simulink model "compute_control"  (R2020a)
settings: Solver=VariableStepAuto  StartTime=0.0  StopTime=0.7  RelTol=1e-3
values from neighbouring files (symbols this model uses):
  A = [-b_cv/Je, 0, -k/Je;     -b_cv/Je+b_ck/Jeq, -b_ck/Jeq, -(k/Je+k/Jeq);     0 0 0]    [Parameters.m]
  B = [0;0;1]    [Parameters.m]
  Gamma = Bd*d    [Parameters.m]
  Q = [0, 0,    0;     0,  50000, 0;     0,  0,    0]    [Parameters.m]
  R = 1    [Parameters.m]
settings Model: Creator=andre  LastModifiedBy=andre

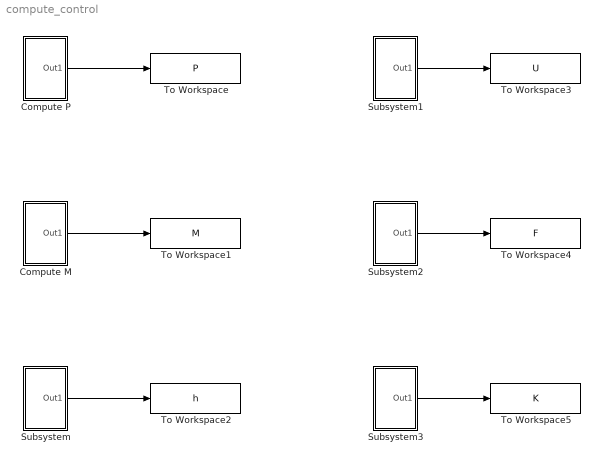
== system compute_control ==
  Compute M : Subsystem
  Compute P : Subsystem
  Subsystem : Subsystem
  Subsystem1 : Subsystem
  Subsystem2 : Subsystem
  Subsystem3 : Subsystem
  To Workspace : ToWorkspace  VariableName=P  SampleTime=-1
  To Workspace1 : ToWorkspace  VariableName=M  SampleTime=-1
  To Workspace2 : ToWorkspace  VariableName=h  SampleTime=-1
  To Workspace3 : ToWorkspace  VariableName=U  SampleTime=-1
  To Workspace4 : ToWorkspace  VariableName=F  SampleTime=-1
  To Workspace5 : ToWorkspace  VariableName=K  SampleTime=-1
  wires:
  Compute P/1(Out1) -> To Workspace/1
  Compute M/1(Out1) -> To Workspace1/1
  Subsystem/1(Out1) -> To Workspace2/1
  Subsystem1/1(Out1) -> To Workspace3/1
  Subsystem2/1(Out1) -> To Workspace4/1
  Subsystem3/1(Out1) -> To Workspace5/1

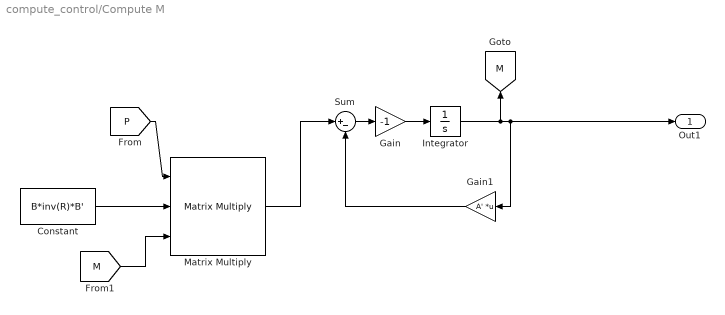
== system compute_control/Compute M ==
  Constant : Constant  Value=B*inv(R)*B'
  Gain : Gain  Gain=-1
  Gain1 : Gain  Gain=A'  Multiplication=Matrix(K*u)
  Integrator : Integrator  InitialCondition=[0;1;0]
  Matrix Multiply : Product  Inputs=3  Multiplication=Matrix(*)
  Sum : Sum  Inputs=|+-
  Out1 : Outport
  tag scope: M=global
  wires:
  [P] -> Matrix Multiply/1
  Gain1/1 -> Sum/2
  Sum/1 -> Gain/1
  Gain/1 -> Integrator/1
  Matrix Multiply/1 -> Sum/1
  Constant/1 -> Matrix Multiply/2
  Integrator/1 -> [M], Out1/1, Gain1/1
  [M] -> Matrix Multiply/3

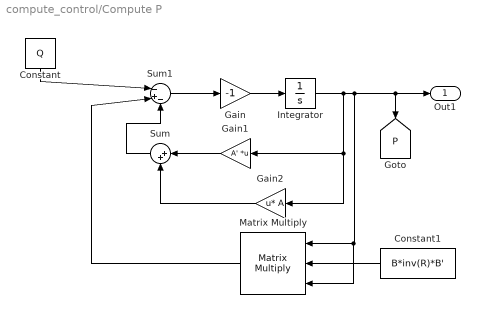
== system compute_control/Compute P ==
  Constant : Constant  Value=Q
  Constant1 : Constant  Value=B*inv(R)*B'
  Gain : Gain  Gain=-1
  Gain1 : Gain  Gain=A'  Multiplication=Matrix(K*u)
  Gain2 : Gain  Gain=A  Multiplication=Matrix(u*K)
  Integrator : Integrator  InitialCondition=zeros(3,3)
  Matrix Multiply : Product  Inputs=3  Multiplication=Matrix(*)
  Sum : Sum  Inputs=|++
  Sum1 : Sum  Inputs=|-+-
  Out1 : Outport
  tag scope: P=global
  wires:
  Sum/1 -> Sum1/3
  Integrator/1 -> Gain1/1, Gain2/1, [P], Out1/1, Matrix Multiply/3, Matrix Multiply/1
  Sum1/1 -> Gain/1
  Constant/1 -> Sum1/1
  Gain/1 -> Integrator/1
  Gain2/1 -> Sum/2
  Gain1/1 -> Sum/1
  Matrix Multiply/1 -> Sum1/2
  Constant1/1 -> Matrix Multiply/2

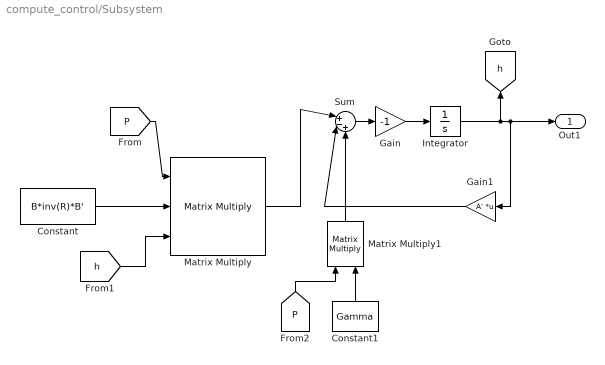
== system compute_control/Subsystem ==
  Constant : Constant  Value=B*inv(R)*B'
  Constant1 : Constant  Value=Gamma
  Gain : Gain  Gain=-1
  Gain1 : Gain  Gain=A'  Multiplication=Matrix(K*u)
  Integrator : Integrator  InitialCondition=[0;0;0]
  Matrix Multiply : Product  Inputs=3  Multiplication=Matrix(*)
  Matrix Multiply1 : Product  Multiplication=Matrix(*)
  Sum : Sum  Inputs=|+-+
  Out1 : Outport
  tag scope: h=global
  wires:
  [h] -> Matrix Multiply/3
  Constant/1 -> Matrix Multiply/2
  Integrator/1 -> [h], Out1/1, Gain1/1
  Gain/1 -> Integrator/1
  Sum/1 -> Gain/1
  Gain1/1 -> Sum/2
  [P] -> Matrix Multiply1/1
  Matrix Multiply/1 -> Sum/1
  [P] -> Matrix Multiply/1
  Matrix Multiply1/1 -> Sum/3
  Constant1/1 -> Matrix Multiply1/2

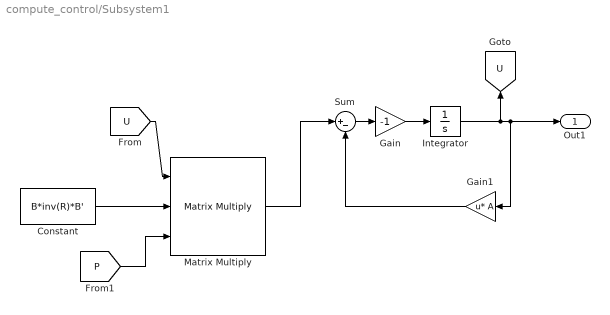
== system compute_control/Subsystem1 ==
  Constant : Constant  Value=B*inv(R)*B'
  Gain : Gain  Gain=-1
  Gain1 : Gain  Gain=A  Multiplication=Matrix(u*K)
  Integrator : Integrator  InitialCondition=[0 1 0]
  Matrix Multiply : Product  Inputs=3  Multiplication=Matrix(*)
  Sum : Sum  Inputs=|+-
  Out1 : Outport
  tag scope: U=global
  wires:
  Gain/1 -> Integrator/1
  Gain1/1 -> Sum/2
  Matrix Multiply/1 -> Sum/1
  Constant/1 -> Matrix Multiply/2
  [P] -> Matrix Multiply/3
  Sum/1 -> Gain/1
  Integrator/1 -> [U], Out1/1, Gain1/1
  [U] -> Matrix Multiply/1

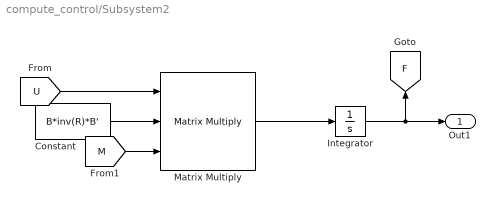
== system compute_control/Subsystem2 ==
  Constant : Constant  Value=B*inv(R)*B'
  Integrator : Integrator
  Matrix Multiply : Product  Inputs=3  Multiplication=Matrix(*)
  Out1 : Outport
  tag scope: F=global
  wires:
  Integrator/1 -> Out1/1, [F]
  Matrix Multiply/1 -> Integrator/1
  [U] -> Matrix Multiply/1
  Constant/1 -> Matrix Multiply/2
  [M] -> Matrix Multiply/3

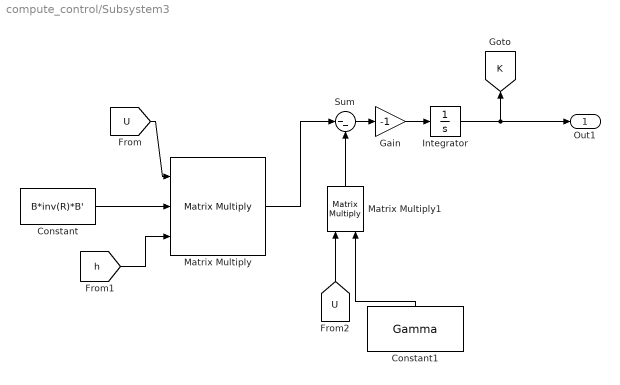
== system compute_control/Subsystem3 ==
  Constant : Constant  Value=B*inv(R)*B'
  Constant1 : Constant  Value=Gamma
  Gain : Gain  Gain=-1
  Integrator : Integrator
  Matrix Multiply : Product  Inputs=3  Multiplication=Matrix(*)
  Matrix Multiply1 : Product  Multiplication=Matrix(*)
  Sum : Sum  Inputs=|--
  Out1 : Outport
  tag scope: K=global
  wires:
  Constant/1 -> Matrix Multiply/2
  [U] -> Matrix Multiply1/1
  Sum/1 -> Gain/1
  Integrator/1 -> Out1/1, [K]
  Matrix Multiply1/1 -> Sum/2
  [h] -> Matrix Multiply/3
  [U] -> Matrix Multiply/1
  Constant1/1 -> Matrix Multiply1/2
  Gain/1 -> Integrator/1
  Matrix Multiply/1 -> Sum/1
